simulink model "Simulink_test_SFunction"  (R2022b)
settings: Solver=FixedStepAuto  StartTime=0.0  StopTime=500  FixedStep=0.10  RelTol=1e-3
values from neighbouring files (symbols this model uses):
  D1 = W2_newnew(x0)    [main_S_F.m]
  D2 = W3_newnew(x0)    [main_S_F.m]
  x0 = [0;-45;pi/2;0;0;-30;0;0;10;0]    [main_S_F.m]
settings Model: Creator=user  LastModifiedBy=user

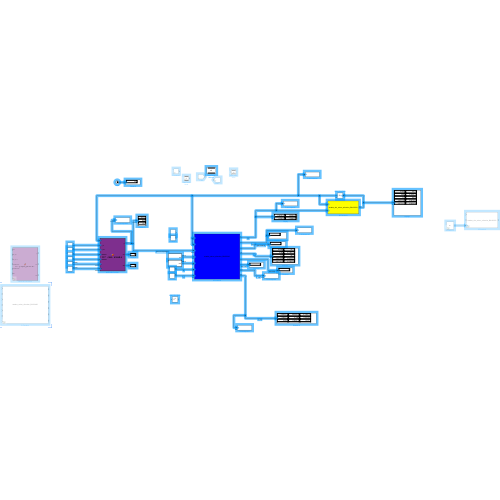
[thumbnail: Simulink's stored preview of the top-level diagram]
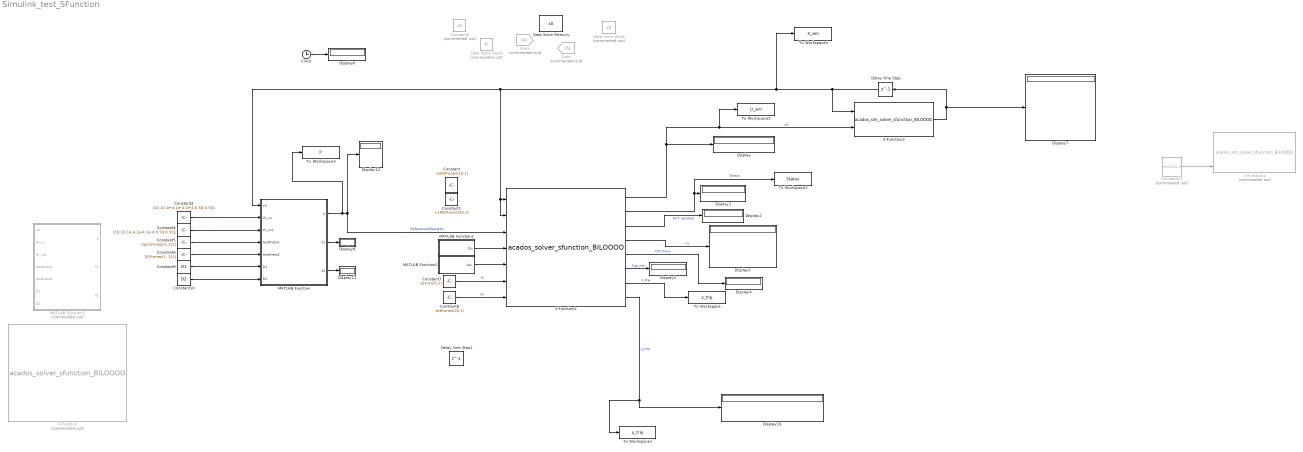
== system Simulink_test_SFunction ==
  Clock : Clock
  Constant : Constant  Value=-1000*ones(10,1)
  Constant1 : Constant  Value=+1000*ones(10,1)
  Constant10 : Constant  Value=D2
  Constant11 : Constant  Commented=on  Value=zeros(24,1)
  Constant2 : Constant  Commented=on  Value=x0
  Constant3 : Constant  Value=[10;10;1e-4;1e-4;1e-4;0.50;0.50];
  Constant4 : Constant  Value=[10;10;1e-4;1e-4;1e-4;0.50;0.50];
  Constant5 : Constant  Value=[(pi/2)*ones(1,21)]
  Constant6 : Constant  Value=[(0)*ones(1, 21)]
  Constant7 : Constant  Value=zeros(20,1)
  Constant8 : Constant  Value=1e8*ones(20,1)
  Constant9 : Constant  Value=D1
  Data Store Memory : DataStoreMemory  DataStoreName=x0  WriteAfterWriteMsg=warning  InitialValue=[0;-45;pi/2;0;0;-30;0;0;10;0]  ShowAdditionalParam=off
  Data Store Read : DataStoreRead  Commented=on  DataStoreName=x0  IndexOptions=Index vector (dialog)  Indices=1  OutputSizes=1
  Data Store Write : DataStoreWrite  Commented=on  DataStoreName=x0  IndexOptions=Index vector (dialog)  Indices=1  OutputSizes=1
  Delay One Step : Delay  DelayLength=1  InitialCondition=x0
  Delay One Step1 : Delay  DelayLength=1  InitialCondition=x0
  Display{,1..8,10..12} (12 alike) : Display
  From : From  Commented=on
  Goto : Goto  Commented=on
  MATLAB Function : MATLAB Function  TreatAsAtomicUnit=on
  MATLAB Function1 : MATLAB Function  TreatAsAtomicUnit=on
  MATLAB Function2 : MATLAB Function  TreatAsAtomicUnit=on
  MATLAB Function3 : MATLAB Function  Commented=on  TreatAsAtomicUnit=on
  S-Function : S-Function  Commented=on  FunctionName=acados_solver_sfunction_BILOOOO  SFunctionDeploymentMode=off  EnableBusSupport=off
  S-Function1 : S-Function  Commented=on  FunctionName=acados_sim_solver_sfunction_BILOOOO  SFunctionDeploymentMode=off  EnableBusSupport=off
  S-Function2 : S-Function  FunctionName=acados_solver_sfunction_BILOOOO  SFunctionDeploymentMode=off  EnableBusSupport=off
  S-Function3 : S-Function  FunctionName=acados_sim_solver_sfunction_BILOOOO  SFunctionDeploymentMode=off  EnableBusSupport=off
  To Workspace : ToWorkspace  VariableName=x_traj  SampleTime=-1
      settings: Save2DSignal=2-D array (concatenate along first dimension)
  To Workspace1 : ToWorkspace  VariableName=u_traj  SampleTime=-1
      settings: Save2DSignal=2-D array (concatenate along first dimension)
  To Workspace2 : ToWorkspace  VariableName=Status  SampleTime=-1
      settings: Save2DSignal=2-D array (concatenate along first dimension)
  To Workspace3 : ToWorkspace  VariableName=P  SaveFormat=Timeseries  SampleTime=-1
      settings: Save2DSignal=2-D array (concatenate along first dimension)
  To Workspace4 : ToWorkspace  VariableName=X_sim  SaveFormat=Structure With Time  SampleTime=-1
  To Workspace5 : ToWorkspace  VariableName=U_sim  SaveFormat=Structure With Time  SampleTime=-1
  wires:
  Constant3/1 -> MATLAB Function/2(W_xu)
  Constant4/1 -> MATLAB Function/3(W_xu1)
  MATLAB Function/1(p) -> To Workspace3/1, Display12/1, S-Function2/3  "References|Weights"
  MATLAB Function1/1(lbu) -> S-Function2/4
  MATLAB Function2/1(ubu) -> S-Function2/5
  Constant7/1 -> S-Function2/6  "lh"
  Constant8/1 -> S-Function2/7  "uh"
  S-Function2/1 -> Display/1, To Workspace5/1, S-Function3/2  "u0"
  S-Function2/2 -> To Workspace2/1, Display1/1  "Status"
  S-Function2/3 -> Display2/1  "KKT residual"
  S-Function2/4 -> Display3/1  "x1"
  S-Function2/5 -> Display4/1  "CPU time"
  S-Function2/6 -> Display5/1  "Sqp_iter"
  Constant9/1 -> MATLAB Function/6(D1)
  Constant10/1 -> MATLAB Function/7(D2)
  Clock/1 -> Display6/1
  S-Function3/1 -> Delay One Step/1, Display7/1
  Delay One Step/1 -> S-Function3/1, To Workspace4/1, S-Function2/2, S-Function2/1, MATLAB Function/1(x0)
  S-Function2/7 -> To Workspace/1  "x_traj"
  S-Function2/8 -> To Workspace1/1, Display10/1  "u_traj"
  Constant11/1 -> S-Function1/3
  Constant5/1 -> MATLAB Function/4(testtheta1)
  Constant6/1 -> MATLAB Function/5(testtheta2)
  MATLAB Function/2(S1) -> Display8/1
  MATLAB Function/3(S2) -> Display11/1

== matlab function Simulink_test_SFunction/MATLAB Function1 ==
  data: lbu output
function lbu = LBU
% Define lower bounds for control inputs
lbu_control = [-11.5; -1; -11.5; -1]; % Control inputs

% Determine how many times to repeat the control bounds
num_repeats = ceil(80 / length(lbu_control)); % Calculate how many times to repeat
lbu = repmat(lbu_control, num_repeats, 1); % Repeat to create a long enough array
lbu = lbu(1:80); % Truncate to exactly 80 elements

% Check size
assert(length(lbu) == 80, 'Lower bounds array must have 80 elements.');

end

== matlab function Simulink_test_SFunction/MATLAB Function ==
  data: x0 input; p output; W_xu input; W_xu1 input; testtheta1 input; testtheta2 input; D1 input; D2 input; S1 output; S2 output
function [p, S1, S2] = OCP_prepare_parameters(x0, W_xu, W_xu1, testtheta1, testtheta2, D1, D2)
    nx = length(x0);
    nu = 4;
    ocp_N = 20; % Number of prediction steps
    % Initialize the parameter array
    p = zeros(504, 1); % 504 elements as per your structure

    % Prepare reference points
    current_state1 = x0(1:2); % Use the updated x0 for car 1
    current_state2 = x0(6:7); % Use the updated x0 for car 2
    
    closest_idx1 = findClosestPoint(current_state1, D1);
    closest_idx2 = findClosestPoint(current_state2, D2);
    
    % Reference points for car 1
    if closest_idx1 + ocp_N <= size(D1, 2)
        reference_points1 = D1(:, closest_idx1:closest_idx1 + ocp_N);
    else
        remaining_points1 = size(D1, 2) - closest_idx1 + 1;
        reference_points1 = D1(:, closest_idx1:end);
        additional_points1 = (ocp_N + 1) - remaining_points1;

        last_x1 = D1(1, end);
        last_y1 = D1(2, end);
        new_x1 = last_x1 - (1:additional_points1) * 0.1; % Assuming 0.1m per step
        new_y1 = last_y1 * ones(1, additional_points1);

        extended_points1 = [new_x1; new_y1];
        reference_points1 = [reference_points1, extended_points1];
    end
    
    % Reference points for car 2
    if closest_idx2 + ocp_N <= size(D2, 2)
        reference_points2 = D2(:, closest_idx2:closest_idx2 + ocp_N);
    else
        remaining_points2 = size(D2, 2) - closest_idx2 + 1;
        reference_points2 = D2(:, closest_idx2:end);
        additional_points2 = (ocp_N + 1) - remaining_points2;

        last_x2 = D2(1, end);
        last_y2 = D2(2, end);
        new_x2 = last_x2 + (1:additional_points2) * 0.1; % Assuming 0.1m per step
        new_y2 = last_y2 * ones(1, additional_points2);

        extended_points2 = [new_x2; new_y2];
        reference_points2 = [reference_points2, extended_points2];
    end

    % Create x_traj_init with the specified structure
    x_traj_init = [
        reference_points1; % x1, y1, ...
        testtheta1';       % theta1
        zeros(1, ocp_N + 1); % v1
        zeros(1, ocp_N + 1); % s1
        reference_points2; % x2, y2, ...
        testtheta2';       % theta2
        zeros(1, ocp_N + 1); % v2
        zeros(1, ocp_N + 1)  % s2
    ];

    % Check sizes
    S1 = size(x_traj_init, 1); % Number of rows
    S2 = size(x_traj_init, 2); % Number of columns

%     % Ensure that x_traj_init has enough rows
%     if S1 < 20
%         error('x_traj_init does not have enough rows. Current size: %d', S1);
%     end

    % Fill the parameter array with references and weights
    for jj = 0:ocp_N
        % Fill references for the first car
        p((jj) * (10 + 14) + 1:(jj) * (10 + 14) + 5) = x_traj_init(1:5, jj + 1); % Ref for car 1
        
        % Fill references for the second car
        p((jj) * (10 + 14) + 6:(jj) * (10 + 14) + 10) = x_traj_init(6:10, jj + 1); % Ref for car 2
        
        % Fill weights for the first car
        p((jj) * (10 + 14) + 11:(jj) * (10 + 14) + 15) = W_xu1(1:5); % Weights for car 1
        
        % Fill weights for the second car
        p((jj) * (10 + 14) + 16:(jj) * (10 + 14) + 20) = W_xu(1:5); % Weights for car 2
        
        % Fill weights for the control inputs
        p((jj) * (10 + 14) + 21:(jj) * (10 + 14) + 24) = [W_xu(6:7);W_xu1(6:7)]; % Control input weights (4 elements)
    end

    % Check if the size of p is correct
    assert(length(p) == 504, 'Parameter array must have 504 elements.');

    % Output parameter array
end

== matlab function Simulink_test_SFunction/MATLAB Function2 ==
  data: ubu output
function ubu = UBU
% Define lower bounds for control inputs
ubu_control = [+11.5; 1; 11.5; 1]; % Control inputs

% Determine how many times to repeat the control bounds
num_repeats = ceil(80 / length(ubu_control)); % Calculate how many times to repeat
ubu = repmat(ubu_control, num_repeats, 1); % Repeat to create a long enough array
ubu = ubu(1:80); % Truncate to exactly 80 elements

% Check size
assert(length(ubu) == 80, 'Lower bounds array must have 80 elements.');

end

== matlab function Simulink_test_SFunction/MATLAB Function3 ==
  data: x0 input; p output; W_xu input; W_xu1 input; testtheta1 input; testtheta2 input; D1 input; D2 input; S1 output; S2 output
function [p,S1,S2] = OCP_prepare_parameters(x0, W_xu, W_xu1, testtheta1, testtheta2,D1,D2)
    nx = length(x0);
    nu = 4;
    ocp_N = 20; % Number of prediction steps
    % Initialize the parameter array
    p = zeros(504, 1); % 504 elements as per your structure
    %%
%     D1=W2_newnew(x0);D2=W3_newnew(x0); %% referencing    needs to be change eventually
    %%
    % Prepare reference points
    current_state1 = x0(1:2); % Use the updated x0
    current_state2 = x0(6:7);
    
    closest_idx1 = findClosestPoint(current_state1, D1);
    closest_idx2 = findClosestPoint(current_state2, D2);
    
    % Reference points for car 1
    if closest_idx1 + ocp_N <= size(D1, 2)
        reference_points1 = D1(:, closest_idx1:closest_idx1+ocp_N);
    else
        remaining_points1 = size(D1, 2) - closest_idx1 + 1;
        reference_points1 = D1(:, closest_idx1:end);
        additional_points1 = (ocp_N + 1) - remaining_points1;
        
        last_x1 = D1(1, end);
        last_y1 = D1(2, end);
        new_x1 = last_x1 - (1:additional_points1) * 0.1; % Assuming 0.1m per step
        new_y1 = last_y1 * ones(1, additional_points1);
        
        extended_points1 = [new_x1; new_y1];
        reference_points1 = [reference_points1, extended_points1];
    end
    
    % Reference points for car 2
    if closest_idx2 + ocp_N <= size(D2, 2)
        reference_points2 = D2(:, closest_idx2:closest_idx2+ocp_N);
    else
        remaining_points2 = size(D2, 2) - closest_idx2 + 1;
        reference_points2 = D2(:, closest_idx2:end);
        additional_points2 = (ocp_N + 1) - remaining_points2;

        last_x2 = D2(1, end);
        last_y2 = D2(2, end);
        new_x2 = last_x2 + (1:additional_points2) * 0.1; % Assuming 0.1m per step
        new_y2 = last_y2 * ones(1, additional_points2);
        
        extended_points2 = [new_x2; new_y2];
        reference_points2 = [reference_points2, extended_points2];
    end
    
    % Combine reference points and prepare parameter vector
    x_traj_init = [reference_points1; testtheta1'; zeros(1, ocp_N + 1); zeros(1, ocp_N + 1);reference_points2; testtheta2'; zeros(1, ocp_N + 1); zeros(1, ocp_N + 1)];

    S1=size(x_traj_init,1);
    S2=size(x_traj_init,2);
    
    % Fill the parameter array
    for jj = 1:ocp_N
        p((jj - 1) * nx + 1:jj * nx) = x_traj_init(:, jj);
    end
    
    % Weights - example, adapt as needed
    p(nx*ocp_N + 1:nx*ocp_N + 14) = [W_xu1(1:5); W_xu(1:5); W_xu1(6:7); W_xu(6:7)];

%     % Check if the size of p is correct
%     assert(length(p) == 504, 'Parameter array must have 504 elements.');

    % Output parameter array
end
